simulink model "Sim"  (R2022a)
settings: Solver=FixedStepAuto  StartTime=0.0  StopTime=10  FixedStep=0.01  RelTol=1e-3
values from neighbouring files (symbols this model uses):
  vo = 0.1    [Parametros.m]
  xa = 39.5/1000    (= 0.0395)    [Parametros.m]
libraries: slpidlib x1, cstblocks x1
settings Model: Creator=Francisco  LastModifiedBy=Francisco

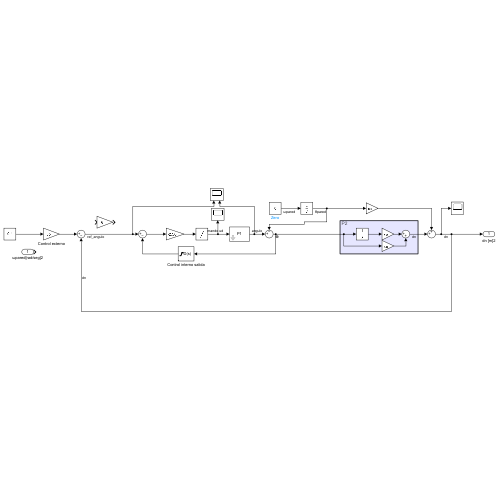
[thumbnail: Simulink's stored preview of the top-level diagram]
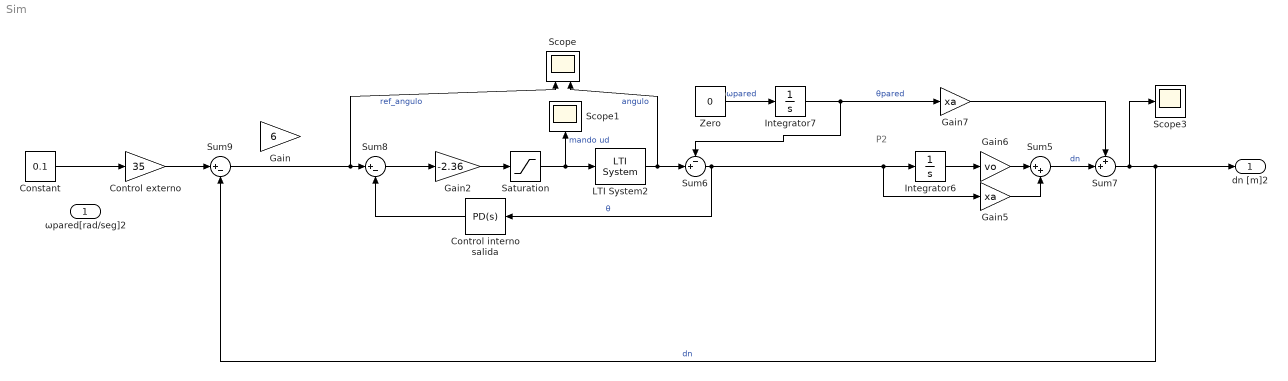
== system Sim ==
  note: P2
  ωpared[rad/seg]2 : Inport
  Constant : Constant  Value=0.1
  Control externo : Gain  Gain=35
  Control interno salida : slpidlib/PID Controller  Controller=PD  Form=Ideal  TimeDomain=Continuous-time  UseExternalTs=off  SampleTime=-1  IntegratorMethod=Forward Euler  FilterMethod=Forward Euler  ControllerParametersSource=internal  P=-2.36  I=3.51415558056919  UseKiTs=on  D=0.166  N=54.2169  UseFilter=on  TunerSelectOption=Transfer Function Based (PID Tuner App)  InitialConditionSource=internal  InitialConditionForIntegrator=0.2  InitialConditionForFilter=0  DifferentiatorICPrevScaledInput=0  ExternalReset=none  TrackingMode=off  Kt=1  LimitOutput=on  SatLimitsSource=internal  UpperSaturationLimit=100  LowerSaturationLimit=-100  LinearizeAsGain=on  AntiWindupMode=clamping  Kb=1  POutMin=[]  POutMax=[]  IOutMin=[]  IOutMax=[]  DOutMin=[]  DOutMax=[]  NOutMin=[]  NOutMax=[]  SumOutMin=[]  SumOutMax=[]  SaturationOutMin=[]  SaturationOutMax=[]  PParamMin=[]  PParamMax=[]  IParamMin=[]  IParamMax=[]  DParamMin=[]  DParamMax=[]  NParamMin=[]  NParamMax=[]  KbParamMin=[]  KbParamMax=[]  KtParamMin=[]  KtParamMax=[]  KbOutMin=[]  KbOutMax=[]  KtOutMin=[]  KtOutMax=[]  IntegratorOutMin=[]  IntegratorOutMax=[]  FilterOutMin=[]  FilterOutMax=[]  SumI1OutMin=[]  SumI1OutMax=[]  SumI2OutMin=[]  SumI2OutMax=[]  SumI3OutMin=[]  SumI3OutMax=[]  SumI4OutMin=[]  SumI4OutMax=[]  SumDOutMin=[]  SumDOutMax=[]  DifferentiatorOutMin=[]  DifferentiatorOutMax=[]  FilterDiffOutCoefMin=[]  FilterDiffOutCoefMax=[]  ReciprocalOutMin=[]  ReciprocalOutMax=[]  SumDenOutMin=[]  SumDenOutMax=[]  SumNumOutMin=[]  SumNumOutMax=[]  DivideOutMin=[]  DivideOutMax=[]  UdiffTsProdOutMin=[]  UdiffTsProdOutMax=[]  NTsProdOutMin=[]  NTsProdOutMax=[]  UintegralTsProdOutMin=[]  UintegralTsProdOutMax=[]  UngainTsProdOutMin=[]  UngainTsProdOutMax=[]  IntegratorContinuousStateAttributes=''  IntegratorStateMustResolveToSignalObject=off  IntegratorRTWStateStorageClass=Auto  FilterContinuousStateAttributes=''  FilterStateMustResolveToSignalObject=off  FilterRTWStateStorageClass=Auto  ParallelPVariant=Passthrough  IdealPVariant=InternalParameters  IVariant=Disabled  DVariant=InternalParameters  IntegratorVariant=Disabled  SatVariant=Enabled  AWVariant=Disabled  PCopyVariant=Disabled  TRVariant=Disabled  FdbkBlocksVariant=Forward  IdealPFdbkVariant=Disabled  SatFdbkVariant=Disabled  DerivativeFilterVariant=ContFilter  NVariant=InternalParameters  NCopyVariant=Disabled  FilterICVariant=InternalICsFilter  IntegratorICVariant=Disabled  ExternalResetVariant=Disabled  TRSumVariant=Passthrough  SumFdbkVariant=Disabled  SumVariant=Sum_PD  TsampFilterVariant=InternalTs  TsampNgainVariant=Passthrough  TsampIntegralVariant=Disabled_SignalSpec  ExternalSaturationOutDataTypeStr=Inherit: Same as second input  aMode=0
  Gain : Gain  Gain=6
  Gain2 : Gain  Gain=-2.36
  Gain5 : Gain  Gain=xa
  Gain6 : Gain  Gain=vo
  Gain7 : Gain  Gain=xa
  Integrator6 : Integrator  InitialCondition=2
  Integrator7 : Integrator
  LTI System2 : cstblocks/LTI System  sys=P1  IC=[]
  Saturation : Saturate  UpperLimit=50  LowerLimit=-50
  Scope : Scope  NumInputPorts=2
  Scope1 : Scope
  Scope3 : Scope
  Sum5 : Sum  Inputs=|++
  Sum6 : Sum  Inputs=-+|
  Sum7 : Sum  Inputs=++|
  Sum8 : Sum  Inputs=|+-
  Sum9 : Sum  Inputs=|+-
  Zero : Constant  Value=0  OutDataTypeStr=Inherit: Inherit via back propagation
  dn [m]2 : Outport
  wires:
  Gain7/1 -> Sum7/1
  Gain6/1 -> Sum5/1
  Gain5/1 -> Sum5/2
  Sum7/1 -> Scope3/1, Sum9/2, dn [m]2/1  "dn"
  Zero/1 -> Integrator7/1  "ωpared"
  Integrator7/1 -> Sum6/1, Gain7/1  "θpared"
  Integrator6/1 -> Gain6/1
  Sum6/1 -> Gain5/1, Integrator6/1, Control interno salida/1  "θ"
  LTI System2/1 -> Scope/2, Sum6/2  "angulo"
  Gain2/1 -> Saturation/1
  Sum5/1 -> Sum7/2  "dn"
  Sum8/1 -> Gain2/1
  Saturation/1 -> LTI System2/1, Scope1/1  "mando ud"
  Sum9/1 -> Scope/1, Sum8/1  "ref_angulo"
  Constant/1 -> Control externo/1
  Control externo/1 -> Sum9/1
  Control interno salida/1 -> Sum8/2
